simulink model "sampleModel290"  (R2021b)
settings: Solver=VariableStepAuto  StartTime=0.0  StopTime=10.0  RelTol=1e-3
undefined symbols (not defined in the file or in its folder): DiscIntNeverNeededParam
libraries: simulink x14, slpidlib x2
settings Model: Creator=user  LastModifiedBy=user

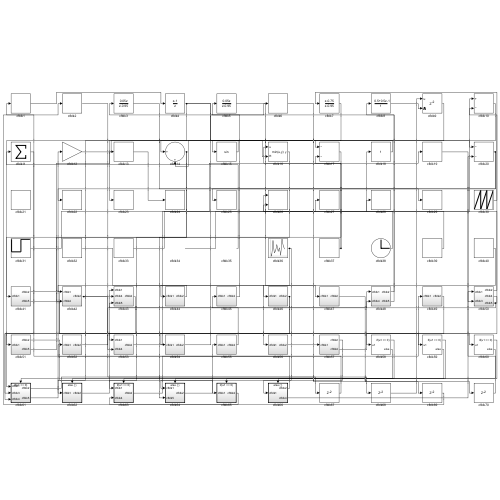
[thumbnail: Simulink's stored preview of the top-level diagram]
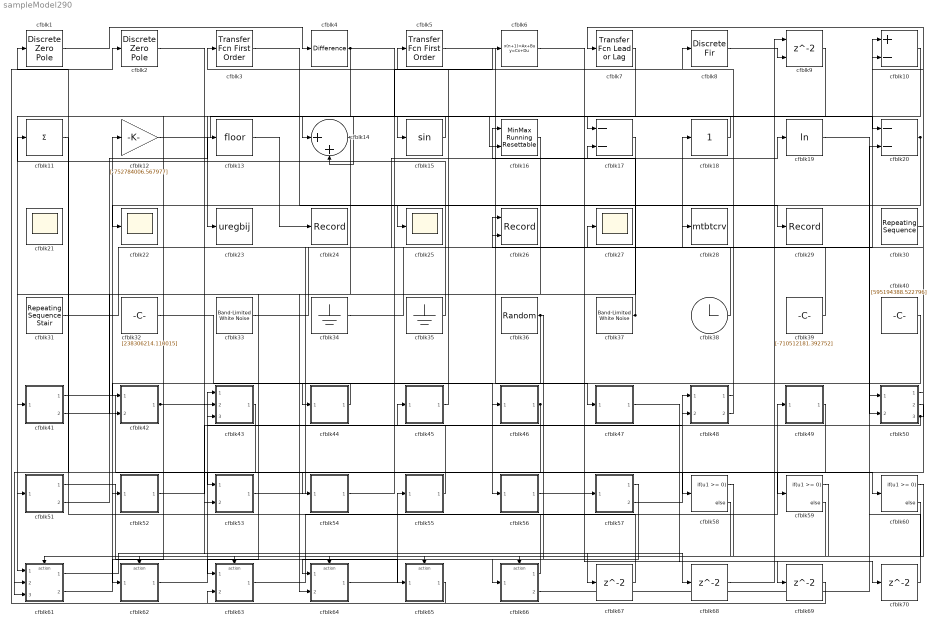
== system sampleModel290 ==
  cfblk1 : DiscreteZeroPole  Poles=[0 0.5]  Gain=1
  cfblk10 : Sum  Inputs=+-
  cfblk11 : Sum  Inputs=+
  cfblk12 : Gain  Gain=[-752784006.567977]
  cfblk13 : Rounding
  cfblk14 : Sum  Inputs=|++
  cfblk15 : Trigonometry
  cfblk16 : simulink/Math Operations/MinMax Running Resettable  Function=min  vinit=0.0
  cfblk17 : Sum  Inputs=--
  cfblk18 : simulink/Math Operations/Slider Gain  gain=1  low=0  high=2
  cfblk19 : Math  Operator=log  SaturateOnIntegerOverflow=on
  cfblk2 : DiscreteZeroPole  Poles=[0 0.5]  Gain=1
  cfblk20 : Sum  Inputs=--
  cfblk{21..22,25,27} (4 alike) : Scope
      cfblk21 settings: Floating=on
  cfblk23 : ToWorkspace  VariableName=uregbij  SaveFormat=Timeseries  SampleTime=-1
  cfblk24 : Record  FileSettingsInternal="{\"entries\":[{\"content\":{\"excelSettings\":{\"content\":{},\"type\":\"Streamout.ExcelSettings\"}},\"type\":\"Streamout.FileSettingStorage\",\"uuid\":\"02e6ebe4-4f75-4483-8c40-05cdad5e9980\"}],\"packageUris\":[\"http://schema.mathworks.com/mf0/streamout_blocks/R2020a\"],\"version\":\"1.0\"}"  SignalsInternal="{\"entries\":[{\"content\":{\"signals\":[{\"content\":{\"blockPath\":[\"sampleModel290/cfblk24\"],\"channel\":[],\"dimensions\":[1],\"domain\":\"sampleModel290/cfblk24\",\"lineColor\":\"#b746ff\",\"plots\":[1],\"port\":1,\"sid\":[\"\"],\"signalID\":12410,\"signalName\":\"cfblk13\"},\"type\":\"RecordBlkView.Signal\",\"uuid\":\"8fecd66d-b984-43b4-8109-c7cccdd95abe\"}]},\"type\":\"RecordBlkView.InputSignals\",\"uuid\":\"a5a1af20-5ce4-4407-aad3-677f96b56cc4\"}],\"packageUris\":[\"http://schema.mathworks.com/mf0/streamout_blocks/R2020a\"],\"version\":\"1.0\"}"  VisualizationBindings="{\"sparklinesplugin\":{\"info\":[{\"bindingParametersList\":[],\"subplotID\":1}]}}"
  cfblk26 : Record  FileSettingsInternal="{\"entries\":[{\"content\":{\"excelSettings\":{\"content\":{},\"type\":\"Streamout.ExcelSettings\"}},\"type\":\"Streamout.FileSettingStorage\",\"uuid\":\"e9eff6ce-7325-488c-8dda-929286e97066\"}],\"packageUris\":[\"http://schema.mathworks.com/mf0/streamout_blocks/R2020a\"],\"version\":\"1.0\"}"  Layout=[1 1]  SignalsInternal="{\"entries\":[{\"content\":{\"signals\":[{\"content\":{\"blockPath\":[\"sampleModel290/cfblk26\"],\"channel\":[],\"dimensions\":[1],\"domain\":\"sampleModel290/cfblk26\",\"lineColor\":\"#a2142f\",\"plots\":[1],\"port\":1,\"sid\":[\"\"],\"signalID\":12398,\"signalName\":\"cfblk39\"},\"type\":\"RecordBlkView.Signal\",\"uuid\":\"f127209e-a6a9-45f0-a171-9e263d700d63\"},{\"content\":{\"blockPath\":[\"sampleModel290/cfblk26\"],\"channel\":[],\"dimensions\":[1],\"domain\":\"sampleModel290/cfblk26\",\"lineColor\":\"#139fff\",\"plots\":[1],\"port\":2,\"sid\":[\"\"],\"signalID\":12402,\"signalName\":\"cfblk50:3\"},\"type\":\"RecordBlkView.Signal\",\"uuid\":\"98f7e693-a703-42fe-986a-2b7354ebe36f\"}]},\"type\":\"RecordBlkView.InputSignals\",\"uuid\":\"39c7099a-60aa-477f-8b96-0c18c85ffd2a\"}],\"packageUris\":[\"http://schema.mathworks.com/mf0/streamout_blocks/R2020a\"],\"version\":\"1.0\"}"  VisualizationBindings="{\"xyplotplugin\":{\"info\":[{\"series\":[{\"bindingParametersList\":[{\"parameter\":\"X-Axis\",\"signalID\":12398,\"signalName\":\"cfblk39\"},{\"parameter\":\"Y-Axis\",\"signalID\":12402,\"signalName\":\"cfblk50:3\"}],\"seriesID\":48777}],\"subplotID\":1}]}}"  CompatibilityTag=XY
  cfblk28 : ToWorkspace  VariableName=mtbtcrv  SaveFormat=Timeseries  SampleTime=-1
  cfblk29 : Record  FileSettingsInternal="{\"entries\":[{\"content\":{\"excelSettings\":{\"content\":{},\"type\":\"Streamout.ExcelSettings\"}},\"type\":\"Streamout.FileSettingStorage\",\"uuid\":\"29b8966b-b4bc-476a-ae5d-9c117f13036d\"}],\"packageUris\":[\"http://schema.mathworks.com/mf0/streamout_blocks/R2020a\"],\"version\":\"1.0\"}"  SignalsInternal="{\"entries\":[{\"content\":{\"signals\":[{\"content\":{\"blockPath\":[\"sampleModel290/cfblk29\"],\"channel\":[],\"dimensions\":[1],\"domain\":\"sampleModel290/cfblk29\",\"lineColor\":\"#ff6929\",\"plots\":[1],\"port\":1,\"sid\":[\"\"],\"signalID\":12406,\"signalName\":\"cfblk3\"},\"type\":\"RecordBlkView.Signal\",\"uuid\":\"751a8cc0-37be-4623-afca-9451bd3e439f\"}]},\"type\":\"RecordBlkView.InputSignals\",\"uuid\":\"efe1f030-47b9-4a82-add3-9ef924c5a613\"}],\"packageUris\":[\"http://schema.mathworks.com/mf0/streamout_blocks/R2020a\"],\"version\":\"1.0\"}"  VisualizationBindings="{\"sparklinesplugin\":{\"info\":[{\"bindingParametersList\":[],\"subplotID\":1}]}}"
  cfblk3 : simulink/Discrete/Transfer Fcn First Order  PoleZ=0.95  ICPrevOutput=0.0  DoSatur=off
  cfblk30 : simulink/Sources/Repeating Sequence  rep_seq_t=[0 2]  rep_seq_y=[-439642906.044889, 580316743.252172]
  cfblk31 : simulink/Sources/Repeating Sequence Stair  OutValues=[-827894639.899098, -721172188.540214]  tsamp=-1  OutMin=[]  OutMax=[]  OutDataTypeStr=double  OutputDataTypeScalingMode=double  OutDataType=fixdt(0,8)  ConRadixGroup=Best Precision: Vector-wise  OutScaling=2^-12
  cfblk32 : Constant  Value=[238306214.110015]  SampleTime=1
  cfblk33 : simulink/Sources/Band-Limited White Noise  Cov=[2286779545.948894]  Ts=0.1  seed=[6396875379.000000]
  cfblk34 : Ground
  cfblk35 : Ground
  cfblk36 : UniformRandomNumber  Minimum=[-8823997467.295820]  Maximum=[646647958.564841]  Seed=[60070097.000000]  SampleTime=0.1
  cfblk37 : simulink/Sources/Band-Limited White Noise  Cov=[6844553857.044216]  Ts=0.1  seed=[8015598396.000000]
  cfblk38 : Clock
  cfblk39 : Constant  Value=[-710512181.392752]  SampleTime=1
  cfblk4 : simulink/Discrete/Difference  ICPrevInput=0.0  OutMin=[]  OutMax=[]  OutDataTypeStr=Inherit: Inherit via back propagation  OutDataType=fixdt(1, 16)  OutScaling=2^-10  DoSatur=off
  cfblk40 : Constant  Value=[595194388.522796]  SampleTime=1
  cfblk41 : Subsystem
  cfblk42 : Subsystem
  cfblk43 : Subsystem
  cfblk44 : Subsystem
  cfblk45 : Subsystem
  cfblk46 : Subsystem
  cfblk47 : Subsystem
  cfblk48 : Subsystem
  cfblk49 : Subsystem
  cfblk5 : simulink/Discrete/Transfer Fcn First Order  PoleZ=0.95  ICPrevOutput=0.0  DoSatur=off
  cfblk50 : Subsystem
  cfblk51 : Subsystem
  cfblk52 : Subsystem
  cfblk53 : Subsystem
  cfblk54 : Subsystem
  cfblk55 : Subsystem
  cfblk56 : Subsystem
  cfblk57 : Subsystem
  cfblk58 : If  IfExpression=u1 >= 0  SampleTime=1
  cfblk59 : If  IfExpression=u1 >= 0  SampleTime=1
  cfblk6 : DiscreteStateSpace
  cfblk60 : If  IfExpression=u1 >= 0  SampleTime=1
  cfblk61 : Subsystem  TreatAsAtomicUnit=on
  cfblk62 : Subsystem  TreatAsAtomicUnit=on
  cfblk63 : Subsystem  TreatAsAtomicUnit=on
  cfblk64 : Subsystem  TreatAsAtomicUnit=on
  cfblk65 : Subsystem  TreatAsAtomicUnit=on
  cfblk66 : Subsystem  TreatAsAtomicUnit=on
  cfblk{67..70} (4 alike) : Delay  SampleTime=1
  cfblk7 : simulink/Discrete/Transfer Fcn Lead or Lag  PoleZ=0.95  ZeroZ=0.75  ICPrevOutput=0.0  ICPrevInput=0.0  DoSatur=off
      settings: SourceProductBaseCode=SL
  cfblk8 : DiscreteFir  SampleTime=1
  cfblk9 : Delay  ShowEnablePort=on  SampleTime=1
      settings: InputPortMap=u0,e6
  wires:
  cfblk13/1 -> cfblk24/1
  cfblk20/1 -> cfblk25/1, cfblk22/1
  cfblk53/1(cfblk2) -> cfblk19/1
  cfblk18/1 -> cfblk61/1(cfblk1)
  cfblk63/1(cfblk2) -> cfblk49/1(cfblk1)
  cfblk65/1(cfblk2) -> cfblk2/1
  cfblk15/1 -> cfblk14/1
  cfblk64/1(cfblk2) -> cfblk55/1(cfblk1)
  cfblk1/1 -> cfblk4/1
  cfblk5/1 -> cfblk47/1(cfblk1)
  cfblk31/1 -> cfblk18/1
  cfblk45/1(cfblk2) -> cfblk5/1
  cfblk43/1(cfblk2) -> cfblk61/2(cfblk3)
  cfblk54/1(cfblk2) -> cfblk6/1
  cfblk62/1(cfblk2) -> cfblk43/1(cfblk1)
  cfblk41/1(cfblk2) -> cfblk60/1
  cfblk40/1 -> cfblk44/1(cfblk1)
  cfblk46/1(cfblk2) -> cfblk61/3(cfblk4), cfblk53/2(cfblk4)
  cfblk56/1(cfblk2) -> cfblk57/1(cfblk1)
  cfblk17/1 -> cfblk41/1(cfblk1)
  cfblk34/1 -> cfblk10/1
  cfblk57/1(cfblk2) -> cfblk64/1(cfblk1)
  cfblk51/1(cfblk2) -> cfblk65/1(cfblk1)
  cfblk9/1 -> cfblk15/1
  cfblk49/1(cfblk2) -> cfblk54/1(cfblk1)
  cfblk33/1 -> cfblk27/1
  cfblk38/1 -> cfblk28/1
  cfblk3/1 -> cfblk29/1
  cfblk36/1 -> cfblk56/1(cfblk1), cfblk66/1(cfblk1)
  cfblk19/1 -> cfblk50/2(cfblk3)
  cfblk30/1 -> cfblk7/1
  cfblk61/2(cfblk5) -> cfblk12/1
  cfblk39/1 -> cfblk26/1
  cfblk4/1 -> cfblk23/1, cfblk17/1, cfblk16/2
  cfblk57/2(cfblk4) -> cfblk48/1(cfblk1)
  cfblk16/1 -> cfblk63/1(cfblk1)
  cfblk12/1 -> cfblk20/1
  cfblk37/1 -> cfblk16/1, cfblk17/2
  cfblk10/1 -> cfblk62/1(cfblk1)
  cfblk41/2(cfblk5) -> cfblk53/1(cfblk1)
  cfblk66/1(cfblk2) -> cfblk52/1(cfblk1)
  cfblk51/2(cfblk5) -> cfblk13/1
  cfblk44/1(cfblk2) -> cfblk42/1(cfblk1)
  cfblk52/1(cfblk2) -> cfblk48/2(cfblk4)
  cfblk14/1 -> cfblk42/2(cfblk4), cfblk64/2(cfblk5)
  cfblk42/1(cfblk2) -> cfblk43/2(cfblk4), cfblk59/1
  cfblk66/2(cfblk4) -> cfblk20/2
  cfblk11/1 -> cfblk51/1(cfblk1)
  cfblk8/1 -> cfblk9/2
  cfblk55/1(cfblk2) -> cfblk43/3(cfblk5)
  cfblk50/1(cfblk2) -> cfblk10/2
  cfblk35/1 -> cfblk11/1
  cfblk32/1 -> cfblk46/1(cfblk1)
  cfblk7/1 -> cfblk14/2
  cfblk48/1(cfblk2) -> cfblk8/1
  cfblk50/2(cfblk4) -> cfblk58/1
  cfblk50/3(cfblk5) -> cfblk26/2, cfblk45/1(cfblk1)
  cfblk48/2(cfblk5) -> cfblk3/1
  cfblk58/1 -> cfblk61/Action
  cfblk58/2 -> cfblk62/Action
  cfblk59/1 -> cfblk63/Action
  cfblk59/2 -> cfblk64/Action
  cfblk60/1 -> cfblk65/Action
  cfblk60/2 -> cfblk66/Action
  cfblk2/1 -> cfblk67/1
  cfblk67/1 -> cfblk1/1
  cfblk61/1(cfblk2) -> cfblk68/1
  cfblk68/1 -> cfblk9/1
  cfblk6/1 -> cfblk69/1
  cfblk69/1 -> cfblk63/2(cfblk4)
  cfblk47/1(cfblk2) -> cfblk70/1
  cfblk70/1 -> cfblk50/1(cfblk1)

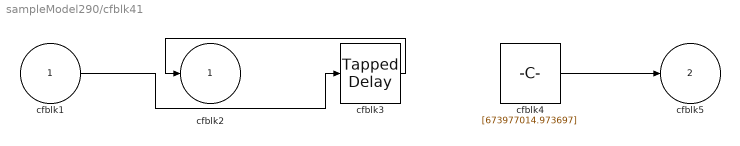
== system sampleModel290/cfblk41 ==
  cfblk1 : Inport
  cfblk3 : simulink/Discrete/Tapped Delay  vinit=0.0  samptime=-1  NumDelays=1  DelayOrder=Oldest  includeCurrent=off
  cfblk4 : Constant  Value=[673977014.973697]  SampleTime=1
  cfblk2 : Outport
  cfblk5 : Outport  Port=2
  wires:
  cfblk4/1 -> cfblk5/1
  cfblk3/1 -> cfblk2/1
  cfblk1/1 -> cfblk3/1

== system sampleModel290/cfblk42 ==
  cfblk1 : Inport
  cfblk4 : Inport  Port=2
  cfblk3 : ComplexToMagnitudeAngle
  cfblk2 : Outport
  wires:
  cfblk1/1 -> cfblk2/1
  cfblk4/1 -> cfblk3/1

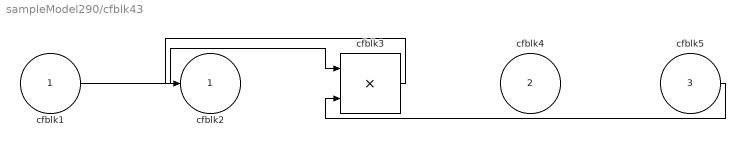
== system sampleModel290/cfblk43 ==
  cfblk1 : Inport
  cfblk4 : Inport  Port=2
  cfblk5 : Inport  Port=3
  cfblk3 : Product  Inputs=**
  cfblk2 : Outport
  wires:
  cfblk1/1 -> cfblk3/1
  cfblk5/1 -> cfblk3/2
  cfblk3/1 -> cfblk2/1

== system sampleModel290/cfblk44 ==
  cfblk1 : Inport
  cfblk3 : UnitDelay  HasFrameUpgradeWarning=on
  cfblk2 : Outport
  wires:
  cfblk1/1 -> cfblk3/1
  cfblk3/1 -> cfblk2/1

== system sampleModel290/cfblk45 ==
  cfblk1 : Inport
  cfblk3 : Sum  Inputs=+-
  cfblk2 : Outport
  wires:
  cfblk3/1 -> cfblk2/1
  cfblk1/1 -> cfblk3/1, cfblk3/2

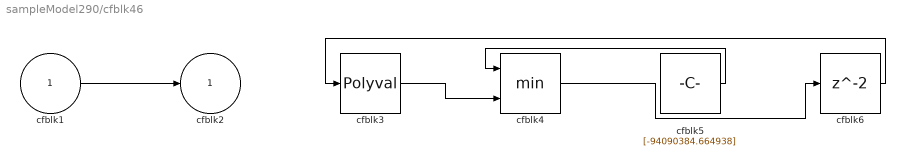
== system sampleModel290/cfblk46 ==
  cfblk1 : Inport
  cfblk3 : Polyval  Coefs=[ +2.081618890e-019, -1.441693666e-014, +4.719686976e-010, -8.536869453e-006, +1.621573104e-001, -8.087801117e+001 ]
  cfblk4 : MinMax  Inputs=2
  cfblk5 : Constant  Value=[-94090384.664938]  SampleTime=1
  cfblk6 : Delay  SampleTime=1
  cfblk2 : Outport
  wires:
  cfblk1/1 -> cfblk2/1
  cfblk5/1 -> cfblk4/1
  cfblk3/1 -> cfblk4/2
  cfblk4/1 -> cfblk6/1
  cfblk6/1 -> cfblk3/1

== system sampleModel290/cfblk47 ==
  cfblk1 : Inport
  cfblk3 : slpidlib/PID Controller (2DOF)  Controller=PID  Form=Parallel  TimeDomain=Discrete-time  UseExternalTs=off  SampleTime=1  IntegratorMethod=Forward Euler  FilterMethod=Forward Euler  ControllerParametersSource=internal  P=1  I=1  D=0  UseFilter=on  N=100  b=1  c=1  TunerSelectOption=Transfer Function Based (PID Tuner App)  InitialConditionSource=internal  InitialConditionForIntegrator=0  InitialConditionForFilter=0  DifferentiatorICPrevScaledInput=0  ExternalReset=none  TrackingMode=off  Kt=1  LimitOutput=off  SatLimitsSource=internal  UpperSaturationLimit=inf  LowerSaturationLimit=-inf  LinearizeAsGain=off  AntiWindupMode=none  Kb=1  POutMin=[]  POutMax=[]  IOutMin=[]  IOutMax=[]  DOutMin=[]  DOutMax=[]  NOutMin=[]  NOutMax=[]  bOutMin=[]  bOutMax=[]  cOutMin=[]  cOutMax=[]  SumOutMin=[]  SumOutMax=[]  SaturationOutMin=[]  SaturationOutMax=[]  PParamMin=[]  PParamMax=[]  IParamMin=[]  IParamMax=[]  DParamMin=[]  DParamMax=[]  NParamMin=[]  NParamMax=[]  bParamMin=[]  bParamMax=[]  cParamMin=[]  cParamMax=[]  KbParamMin=[]  KbParamMax=[]  KtParamMin=[]  KtParamMax=[]  KbOutMin=[]  KbOutMax=[]  KtOutMin=[]  KtOutMax=[]  IntegratorOutMin=[]  IntegratorOutMax=[]  FilterOutMin=[]  FilterOutMax=[]  SumI1OutMin=[]  SumI1OutMax=[]  SumI2OutMin=[]  SumI2OutMax=[]  SumI3OutMin=[]  SumI3OutMax=[]  SumI4OutMin=[]  SumI4OutMax=[]  SumDOutMin=[]  SumDOutMax=[]  Sum1OutMin=[]  Sum1OutMax=[]  Sum2OutMin=[]  Sum2OutMax=[]  Sum3OutMin=[]  Sum3OutMax=[]  DifferentiatorOutMin=[]  DifferentiatorOutMax=[]  FilterDiffOutCoefMin=[]  FilterDiffOutCoefMax=[]  ReciprocalOutMin=[]  ReciprocalOutMax=[]  SumDenOutMin=[]  SumDenOutMax=[]  SumNumOutMin=[]  SumNumOutMax=[]  DivideOutMin=[]  DivideOutMax=[]  UdiffTsProdOutMin=[]  UdiffTsProdOutMax=[]  NTsProdOutMin=[]  NTsProdOutMax=[]  UintegralTsProdOutMin=[]  UintegralTsProdOutMax=[]  UngainTsProdOutMin=[]  UngainTsProdOutMax=[]  IntegratorContinuousStateAttributes=''  IntegratorStateMustResolveToSignalObject=off  IntegratorRTWStateStorageClass=Auto  FilterContinuousStateAttributes=''  FilterStateMustResolveToSignalObject=off  FilterRTWStateStorageClass=Auto  ParallelPVariant=InternalParameters  IdealPVariant=Disabled  IVariant=InternalParameters  DVariant=InternalParameters  bVariant=InternalParameters  cVariant=InternalParameters  IntegratorVariant=Discrete  SatVariant=Disabled  AWVariant=Passthrough  PCopyVariant=Disabled  TRVariant=Disabled  FdbkBlocksVariant=Forward  IdealPFdbkVariant=Disabled  SatFdbkVariant=Disabled  DerivativeFilterVariant=ForwardEulerFilter  NVariant=InternalParameters  NCopyVariant=Disabled  FilterICVariant=InternalICsFilter  IntegratorICVariant=InternalICs  ExternalResetVariant=Disabled  TRSumVariant=Passthrough  SumFdbkVariant=Disabled  SumVariant=Sum_PID  TsampFilterVariant=InternalTs  TsampNgainVariant=Passthrough  TsampIntegralVariant=Passthrough  ExternalSaturationOutDataTypeStr=Inherit: Same as second input
      settings: SourceProductBaseCode=SL
  cfblk2 : Outport
  wires:
  cfblk3/1 -> cfblk2/1
  cfblk1/1 -> cfblk3/1, cfblk3/2

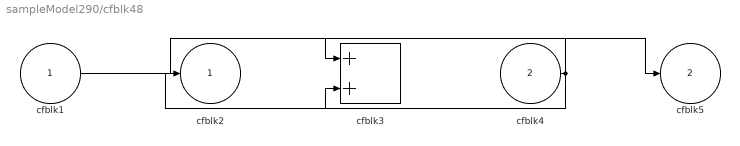
== system sampleModel290/cfblk48 ==
  cfblk1 : Inport
  cfblk4 : Inport  Port=2
  cfblk3 : Sum
  cfblk2 : Outport
  cfblk5 : Outport  Port=2
  wires:
  cfblk1/1 -> cfblk5/1
  cfblk4/1 -> cfblk2/1, cfblk3/1, cfblk3/2

== system sampleModel290/cfblk49 ==
  cfblk1 : Inport
  cfblk3 : Polyval  Coefs=[ +2.081618890e-019, -1.441693666e-014, +4.719686976e-010, -8.536869453e-006, +1.621573104e-001, -8.087801117e+001 ]
  cfblk4 : Constant  Value=[45517312.286219]  SampleTime=1
  cfblk2 : Outport
  wires:
  cfblk4/1 -> cfblk2/1
  cfblk1/1 -> cfblk3/1

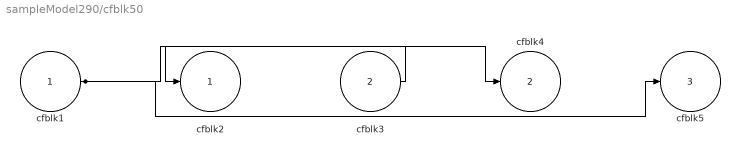
== system sampleModel290/cfblk50 ==
  cfblk1 : Inport
  cfblk3 : Inport  Port=2
  cfblk2 : Outport
  cfblk4 : Outport  Port=2
  cfblk5 : Outport  Port=3
  wires:
  cfblk3/1 -> cfblk2/1
  cfblk1/1 -> cfblk5/1, cfblk4/1

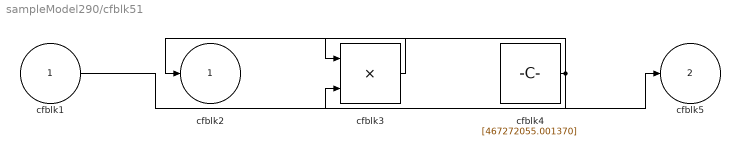
== system sampleModel290/cfblk51 ==
  cfblk1 : Inport
  cfblk3 : Product
  cfblk4 : Constant  Value=[467272055.001370]  SampleTime=1
  cfblk2 : Outport
  cfblk5 : Outport  Port=2
  wires:
  cfblk3/1 -> cfblk2/1
  cfblk1/1 -> cfblk5/1
  cfblk4/1 -> cfblk3/1, cfblk3/2

== system sampleModel290/cfblk52 ==
  cfblk1 : Inport
  cfblk3 : DotProduct  InputSameDT=on  OutDataTypeStr=Inherit: Inherit via internal rule
  cfblk2 : Outport
  wires:
  cfblk1/1 -> cfblk3/1, cfblk3/2
  cfblk3/1 -> cfblk2/1

== system sampleModel290/cfblk53 ==
  cfblk1 : Inport
  cfblk4 : Inport  Port=2
  cfblk3 : simulink/Discrete/Transfer Fcn Real Zero  ZeroZ=0.75  ICPrevInput=0.0  DoSatur=off
      settings: SourceProductBaseCode=SL
  cfblk2 : Outport
  wires:
  cfblk3/1 -> cfblk2/1
  cfblk1/1 -> cfblk3/1

== system sampleModel290/cfblk54 ==
  cfblk1 : Inport
  cfblk3 : simulink/Discrete/Tapped Delay  vinit=0.0  samptime=-1  NumDelays=1  DelayOrder=Oldest  includeCurrent=off
  cfblk2 : Outport
  wires:
  cfblk1/1 -> cfblk2/1, cfblk3/1

== system sampleModel290/cfblk55 ==
  cfblk1 : Inport
  cfblk3 : MinMax
  cfblk2 : Outport
  wires:
  cfblk1/1 -> cfblk3/1
  cfblk3/1 -> cfblk2/1

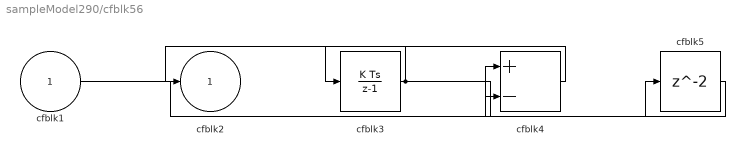
== system sampleModel290/cfblk56 ==
  cfblk1 : Inport
  cfblk3 : DiscreteIntegrator  ICPrevOutput=DiscIntNeverNeededParam  ICPrevScaledInput=DiscIntNeverNeededParam
  cfblk4 : Sum  Inputs=+-
  cfblk5 : Delay  SampleTime=1
  cfblk2 : Outport
  wires:
  cfblk4/1 -> cfblk3/1
  cfblk1/1 -> cfblk4/1
  cfblk3/1 -> cfblk2/1, cfblk5/1
  cfblk5/1 -> cfblk4/2

== system sampleModel290/cfblk57 ==
  cfblk1 : Inport
  cfblk3 : Delay  ShowEnablePort=on  SampleTime=1
      settings: InputPortMap=u0,e6
  cfblk2 : Outport
  cfblk4 : Outport  Port=2
  wires:
  cfblk3/1 -> cfblk2/1
  cfblk1/1 -> cfblk4/1, cfblk3/1, cfblk3/2

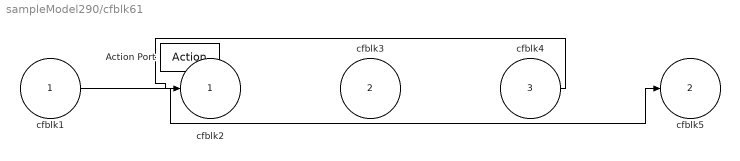
== system sampleModel290/cfblk61 ==
  cfblk1 : Inport
  cfblk3 : Inport  Port=2
  cfblk4 : Inport  Port=3
  Action Port : ActionPort  ActionPortLabel=if(u1 >= 0)
  cfblk2 : Outport
  cfblk5 : Outport  Port=2
  wires:
  cfblk1/1 -> cfblk5/1
  cfblk4/1 -> cfblk2/1

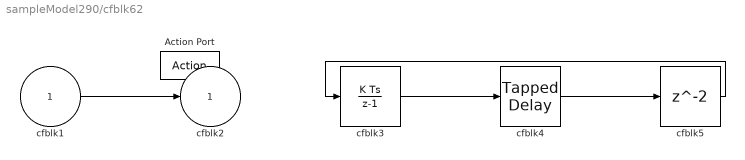
== system sampleModel290/cfblk62 ==
  cfblk1 : Inport
  Action Port : ActionPort  ActionPortLabel=else
  cfblk3 : DiscreteIntegrator  SampleTime=-1  ICPrevOutput=DiscIntNeverNeededParam  ICPrevScaledInput=DiscIntNeverNeededParam
  cfblk4 : simulink/Discrete/Tapped Delay  vinit=0.0  samptime=-1  NumDelays=1  DelayOrder=Oldest  includeCurrent=off
  cfblk5 : Delay
  cfblk2 : Outport
  wires:
  cfblk1/1 -> cfblk2/1
  cfblk3/1 -> cfblk4/1
  cfblk4/1 -> cfblk5/1
  cfblk5/1 -> cfblk3/1

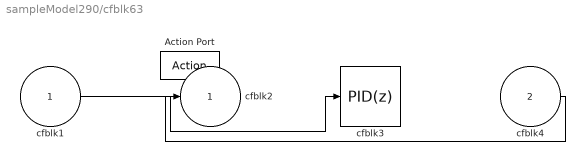
== system sampleModel290/cfblk63 ==
  cfblk1 : Inport
  cfblk4 : Inport  Port=2
  Action Port : ActionPort  ActionPortLabel=if(u1 >= 0)
  cfblk3 : slpidlib/PID Controller  Controller=PID  Form=Parallel  TimeDomain=Discrete-time  UseExternalTs=off  SampleTime=-1  IntegratorMethod=Forward Euler  FilterMethod=Forward Euler  ControllerParametersSource=internal  P=1  I=1  D=0  UseFilter=on  N=100  TunerSelectOption=Transfer Function Based (PID Tuner App)  InitialConditionSource=internal  InitialConditionForIntegrator=0  InitialConditionForFilter=0  DifferentiatorICPrevScaledInput=0  ExternalReset=none  TrackingMode=off  Kt=1  LimitOutput=off  SatLimitsSource=internal  UpperSaturationLimit=inf  LowerSaturationLimit=-inf  LinearizeAsGain=off  AntiWindupMode=none  Kb=1  POutMin=[]  POutMax=[]  IOutMin=[]  IOutMax=[]  DOutMin=[]  DOutMax=[]  NOutMin=[]  NOutMax=[]  SumOutMin=[]  SumOutMax=[]  SaturationOutMin=[]  SaturationOutMax=[]  PParamMin=[]  PParamMax=[]  IParamMin=[]  IParamMax=[]  DParamMin=[]  DParamMax=[]  NParamMin=[]  NParamMax=[]  KbParamMin=[]  KbParamMax=[]  KtParamMin=[]  KtParamMax=[]  KbOutMin=[]  KbOutMax=[]  KtOutMin=[]  KtOutMax=[]  IntegratorOutMin=[]  IntegratorOutMax=[]  FilterOutMin=[]  FilterOutMax=[]  SumI1OutMin=[]  SumI1OutMax=[]  SumI2OutMin=[]  SumI2OutMax=[]  SumI3OutMin=[]  SumI3OutMax=[]  SumI4OutMin=[]  SumI4OutMax=[]  SumDOutMin=[]  SumDOutMax=[]  DifferentiatorOutMin=[]  DifferentiatorOutMax=[]  FilterDiffOutCoefMin=[]  FilterDiffOutCoefMax=[]  ReciprocalOutMin=[]  ReciprocalOutMax=[]  SumDenOutMin=[]  SumDenOutMax=[]  SumNumOutMin=[]  SumNumOutMax=[]  DivideOutMin=[]  DivideOutMax=[]  UdiffTsProdOutMin=[]  UdiffTsProdOutMax=[]  NTsProdOutMin=[]  NTsProdOutMax=[]  UintegralTsProdOutMin=[]  UintegralTsProdOutMax=[]  UngainTsProdOutMin=[]  UngainTsProdOutMax=[]  IntegratorContinuousStateAttributes=''  IntegratorStateMustResolveToSignalObject=off  IntegratorRTWStateStorageClass=Auto  FilterContinuousStateAttributes=''  FilterStateMustResolveToSignalObject=off  FilterRTWStateStorageClass=Auto  ParallelPVariant=InternalParameters  IdealPVariant=Disabled  IVariant=InternalParameters  DVariant=InternalParameters  IntegratorVariant=Discrete  SatVariant=Disabled  AWVariant=Passthrough  PCopyVariant=Disabled  TRVariant=Disabled  FdbkBlocksVariant=Forward  IdealPFdbkVariant=Disabled  SatFdbkVariant=Disabled  DerivativeFilterVariant=ForwardEulerFilter  NVariant=InternalParameters  NCopyVariant=Disabled  FilterICVariant=InternalICsFilter  IntegratorICVariant=InternalICs  ExternalResetVariant=Disabled  TRSumVariant=Passthrough  SumFdbkVariant=Disabled  SumVariant=Sum_PID  TsampFilterVariant=InternalTs  TsampNgainVariant=Passthrough  TsampIntegralVariant=Passthrough  ExternalSaturationOutDataTypeStr=Inherit: Same as second input
  cfblk2 : Outport
  wires:
  cfblk1/1 -> cfblk3/1
  cfblk4/1 -> cfblk2/1

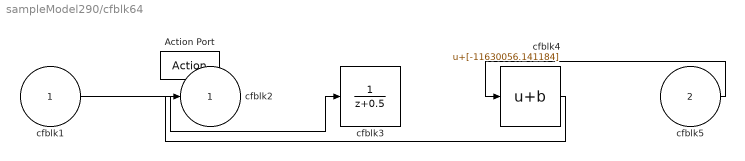
== system sampleModel290/cfblk64 ==
  cfblk1 : Inport
  cfblk5 : Inport  Port=2
  Action Port : ActionPort  ActionPortLabel=else
  cfblk3 : DiscreteTransferFcn
  cfblk4 : Bias  Bias=[-11630056.141184]
  cfblk2 : Outport
  wires:
  cfblk1/1 -> cfblk3/1
  cfblk4/1 -> cfblk2/1
  cfblk5/1 -> cfblk4/1

== system sampleModel290/cfblk65 ==
  cfblk1 : Inport
  Action Port : ActionPort  ActionPortLabel=if(u1 >= 0)
  cfblk3 : Signum
  cfblk4 : Constant  Value=[295531339.054858]  SampleTime=1
  cfblk2 : Outport
  wires:
  cfblk1/1 -> cfblk2/1
  cfblk4/1 -> cfblk3/1

== system sampleModel290/cfblk66 ==
  cfblk1 : Inport
  Action Port : ActionPort  ActionPortLabel=else
  cfblk3 : Delay  DelayLengthSource=Input port
      settings: InputPortMap=u0,p1
  cfblk2 : Outport
  cfblk4 : Outport  Port=2
  wires:
  cfblk1/1 -> cfblk3/1, cfblk3/2
  cfblk3/1 -> cfblk2/1, cfblk4/1
